simulink model "yinji"  (R2023a)
settings: Solver=VariableStepAuto  StartTime=0.0  StopTime=10.0  RelTol=1e-3
settings Model: Creator=Administrator  LastModifiedBy=Administrator

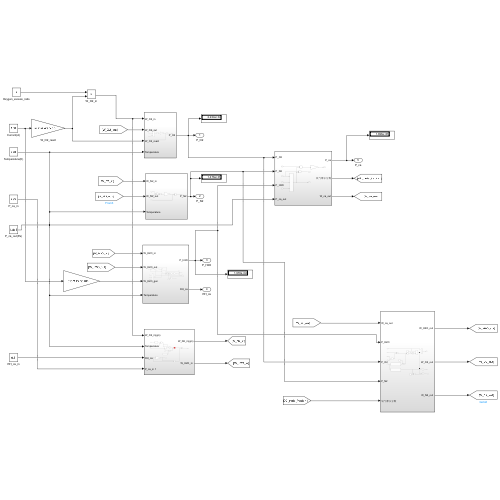
[thumbnail: Simulink's stored preview of the top-level diagram]
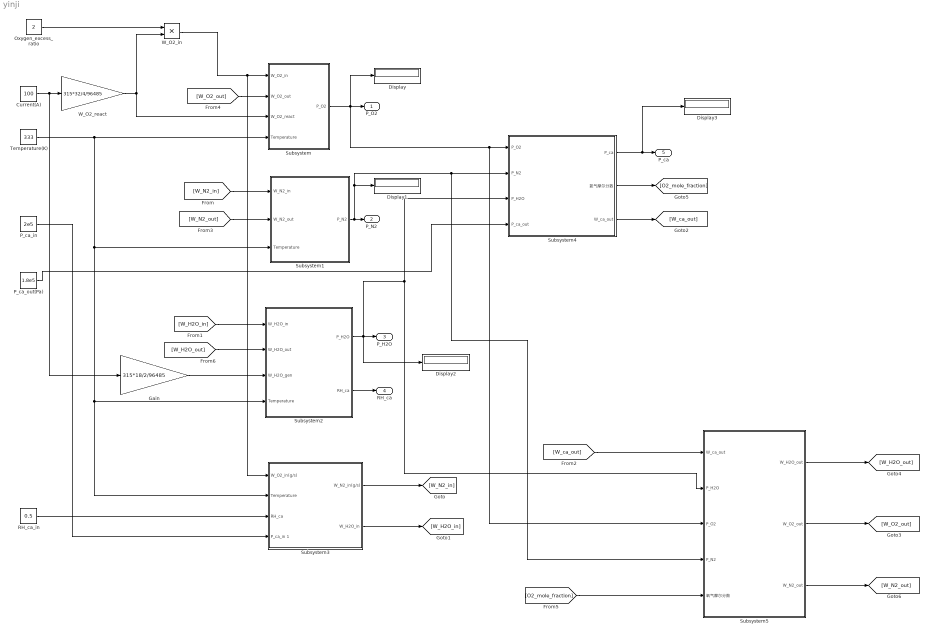
== system yinji ==
  Current(A) : Constant  Value=100
  Display{,1..3} (4 alike) : Display
  Gain : Gain  Gain=315*18/2/96485
  Oxygen_excess_ratio : Constant  Value=2
  P_ca_in : Constant  Value=2e5
  P_ca_out(Pa) : Constant  Value=1.8e5
  RH_ca_in : Constant  Value=0.5
  Subsystem : Subsystem
  Subsystem1 : Subsystem
  Subsystem2 : Subsystem
  Subsystem3 : Subsystem
  Subsystem4 : Subsystem
  Subsystem5 : Subsystem
  Temperature(K) : Constant  Value=333
  W_O2_in : Product
  W_O2_react : Gain  Gain=315*32/4/96485
  P_O2 : Outport
  P_N2 : Outport  Port=2
  P_H2O : Outport  Port=3
  RH_ca : Outport  Port=4
  P_ca : Outport  Port=5
  wires:
  [W_O2_out] -> Subsystem/2(W_O2_out)
  W_O2_react/1 -> W_O2_in/2, Subsystem/3(W_O2_react)
  Current(A)/1 -> Gain/1, W_O2_react/1
  Oxygen_excess_ratio/1 -> W_O2_in/1
  [W_N2_in] -> Subsystem1/1(W_N2_in)
  [W_N2_out] -> Subsystem1/2(W_N2_out)
  [W_H2O_in] -> Subsystem2/1(W_H2O_in)
  [W_H2O_out] -> Subsystem2/2(W_H2O_out)
  Gain/1 -> Subsystem2/3(W_H2O_gen)
  Subsystem2/2(RH_ca) -> RH_ca/1
  W_O2_in/1 -> Subsystem/1(W_O2_in), Subsystem3/1(W_O2_in(g/s))
  Temperature(K)/1 -> Subsystem2/4(Temperature), Subsystem3/2(Temperature), Subsystem1/3(Temperature), Subsystem/4(Temperature)
  RH_ca_in/1 -> Subsystem3/3("RH_ca ")
  P_ca_in/1 -> Subsystem3/4(P_ca_in 1)
  Subsystem3/1(W_N2_in(g/s)) -> [W_N2_in]
  Subsystem3/2("W_H2O_in ") -> [W_H2O_in]
  Subsystem1/1(P_N2) -> Display1/1, Subsystem5/4("P_N2 "), Subsystem4/2("P_N2 "), P_N2/1
  P_ca_out(Pa)/1 -> Subsystem4/4("P_ca_out ")
  Subsystem4/1(P_ca) -> Display3/1, P_ca/1
  Subsystem4/2(氧气摩尔分数) -> [O2_mole_fraction]
  Subsystem4/3(W_ca_out) -> [W_ca_out]
  [W_ca_out] -> Subsystem5/1("W_ca_out ")
  Subsystem2/1(P_H2O) -> Subsystem5/2("P_H2O "), Subsystem4/3("P_H2O "), Display2/1, P_H2O/1
  Subsystem/1(P_O2) -> Display/1, Subsystem5/3("P_O2 "), Subsystem4/1("P_O2 "), P_O2/1
  [O2_mole_fraction] -> Subsystem5/5("氧气摩尔分数 ")
  Subsystem5/1("W_H2O_out ") -> [W_H2O_out]
  Subsystem5/2("W_O2_out ") -> [W_O2_out]
  Subsystem5/3("W_N2_out ") -> [W_N2_out]

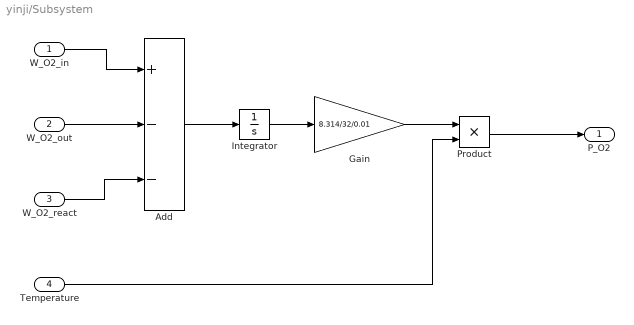
== system yinji/Subsystem ==
  W_O2_in : Inport
  W_O2_out : Inport  Port=2
  W_O2_react : Inport  Port=3
  Temperature : Inport  Port=4
  Add : Sum  Inputs=+--
  Gain : Gain  Gain=8.314/32/0.01
  Integrator : Integrator  InitialCondition=0.01
  Product : Product
  P_O2 : Outport
  wires:
  Temperature/1 -> Product/2
  Integrator/1 -> Gain/1
  Gain/1 -> Product/1
  W_O2_react/1 -> Add/3
  W_O2_in/1 -> Add/1
  Add/1 -> Integrator/1
  Product/1 -> P_O2/1
  W_O2_out/1 -> Add/2

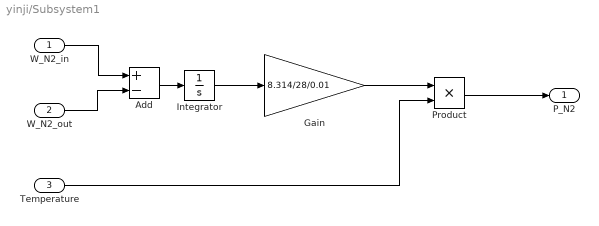
== system yinji/Subsystem1 ==
  W_N2_in : Inport
  W_N2_out : Inport  Port=2
  Temperature : Inport  Port=3
  Add : Sum  Inputs=+-
  Gain : Gain  Gain=8.314/28/0.01
  Integrator : Integrator  InitialCondition=0.01
  Product : Product
  P_N2 : Outport
  wires:
  Temperature/1 -> Product/2
  Integrator/1 -> Gain/1
  Product/1 -> P_N2/1
  Gain/1 -> Product/1
  W_N2_in/1 -> Add/1
  W_N2_out/1 -> Add/2
  Add/1 -> Integrator/1

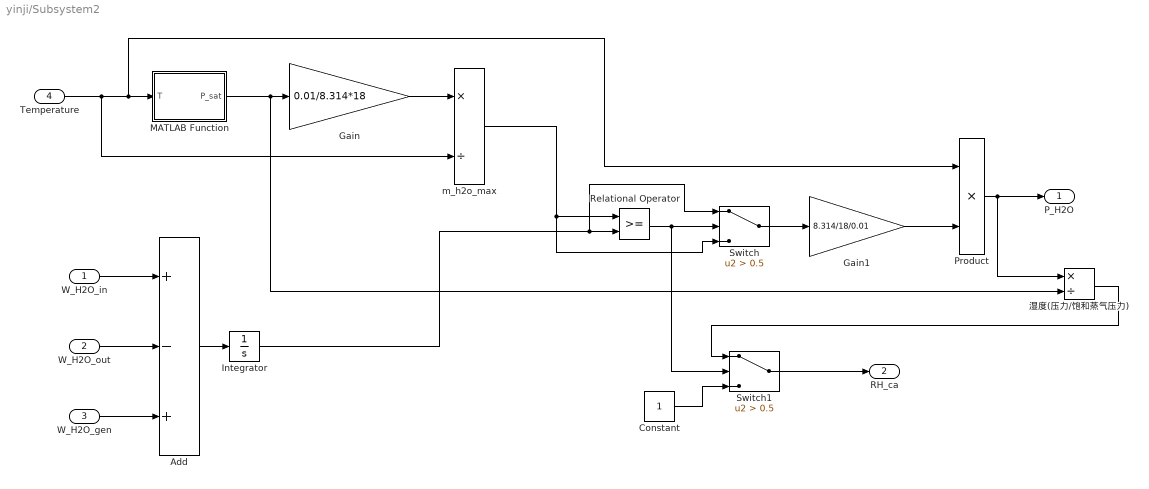
== system yinji/Subsystem2 ==
  W_H2O_in : Inport
  W_H2O_out : Inport  Port=2
  W_H2O_gen : Inport  Port=3
  Temperature : Inport  Port=4
  Add : Sum  Inputs=+-+
  Constant : Constant
  Gain : Gain  Gain=0.01/8.314*18
  Gain1 : Gain  Gain=8.314/18/0.01
  Integrator : Integrator  InitialCondition=0.01
  MATLAB Function : MATLAB Function  TreatAsAtomicUnit=on
  Product : Product
  Relational Operator : RelationalOperator  OutDataTypeStr=boolean  RndMeth=Simplest  InputSameDT=off
  Switch : Switch  Criteria=u2 > Threshold  Threshold=0.5  SaturateOnIntegerOverflow=off  InputSameDT=off
  Switch1 : Switch  Criteria=u2 > Threshold  Threshold=0.5  SaturateOnIntegerOverflow=off  InputSameDT=off
  m_h2o_max : Product  Inputs=*/
  湿度(压力/饱和蒸气压力) : Product  Inputs=*/
  P_H2O : Outport
  RH_ca : Outport  Port=2
  wires:
  湿度(压力/饱和蒸气压力)/1 -> Switch1/1
  Temperature/1 -> m_h2o_max/2, Product/1, MATLAB Function/1(T)
  W_H2O_in/1 -> Add/1
  W_H2O_gen/1 -> Add/3
  W_H2O_out/1 -> Add/2
  Gain1/1 -> Product/2
  Relational Operator/1 -> Switch1/2, Switch/2
  m_h2o_max/1 -> Relational Operator/1, Switch/3
  MATLAB Function/1(P_sat) -> 湿度(压力/饱和蒸气压力)/2, Gain/1
  Integrator/1 -> Switch/1, Relational Operator/2
  Constant/1 -> Switch1/3
  Switch/1 -> Gain1/1
  Add/1 -> Integrator/1
  Product/1 -> P_H2O/1, 湿度(压力/饱和蒸气压力)/1
  Gain/1 -> m_h2o_max/1
  Switch1/1 -> RH_ca/1

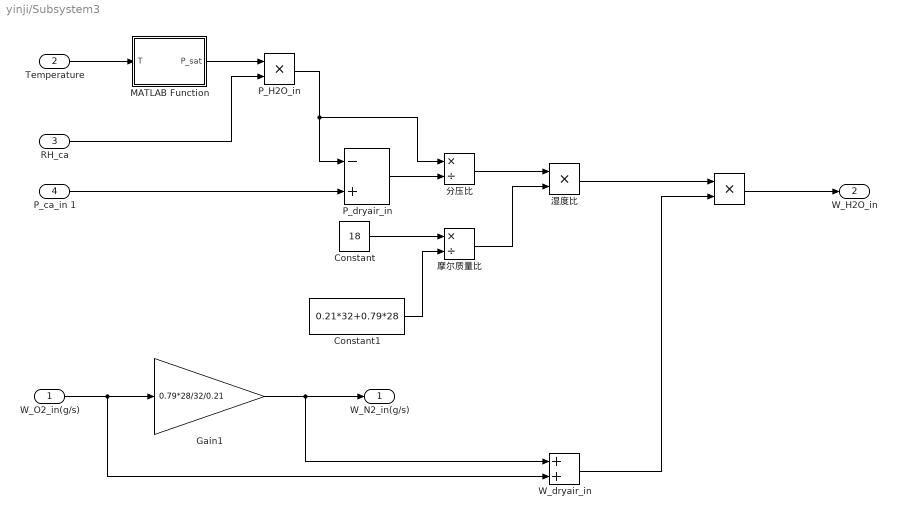
== system yinji/Subsystem3 ==
  W_O2_in(g/s) : Inport
  Temperature : Inport  Port=2
  "RH_ca " : Inport  Port=3
  P_ca_in 1 : Inport  Port=4
  "  " : Product
  Constant : Constant  Value=18
  Constant1 : Constant  Value=0.21*32+0.79*28
  Gain1 : Gain  Gain=0.79*28/32/0.21
  MATLAB Function : MATLAB Function  TreatAsAtomicUnit=on
  P_H2O_in : Product
  P_dryair_in : Sum  Inputs=-+
  W_dryair_in : Sum
  分压比 : Product  Inputs=*/
  摩尔质量比 : Product  Inputs=*/
  湿度比 : Product
  W_N2_in(g/s) : Outport
  "W_H2O_in " : Outport  Port=2
  wires:
  W_O2_in(g/s)/1 -> W_dryair_in/2, Gain1/1
  "  "/1 -> "W_H2O_in "/1
  "RH_ca "/1 -> P_H2O_in/2
  P_dryair_in/1 -> 分压比/2
  MATLAB Function/1(P_sat) -> P_H2O_in/1
  P_H2O_in/1 -> 分压比/1, P_dryair_in/1
  湿度比/1 -> "  "/1
  分压比/1 -> 湿度比/1
  W_dryair_in/1 -> "  "/2
  Temperature/1 -> MATLAB Function/1(T)
  P_ca_in 1/1 -> P_dryair_in/2
  Gain1/1 -> W_N2_in(g/s)/1, W_dryair_in/1
  Constant/1 -> 摩尔质量比/1
  Constant1/1 -> 摩尔质量比/2
  摩尔质量比/1 -> 湿度比/2

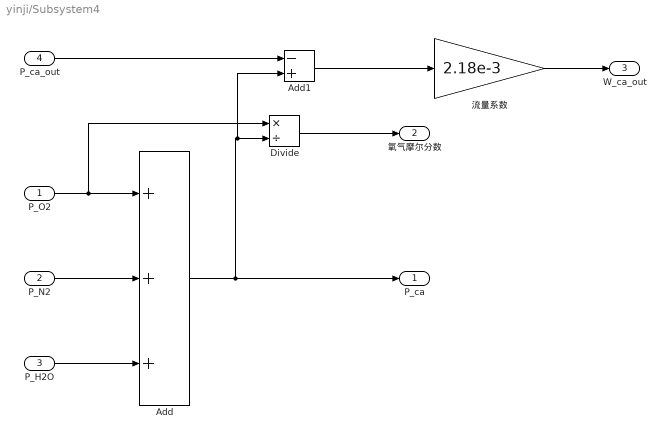
== system yinji/Subsystem4 ==
  "P_O2 " : Inport
  "P_N2 " : Inport  Port=2
  "P_H2O " : Inport  Port=3
  "P_ca_out " : Inport  Port=4
  Add : Sum  Inputs=+++
  Add1 : Sum  Inputs=-+
  Divide : Product  Inputs=*/
  流量系数 : Gain  Gain=2.18e-3
  P_ca : Outport
  氧气摩尔分数 : Outport  Port=2
  W_ca_out : Outport  Port=3
  wires:
  "P_ca_out "/1 -> Add1/1
  "P_O2 "/1 -> Divide/1, Add/1
  Add/1 -> P_ca/1, Add1/2, Divide/2
  Divide/1 -> 氧气摩尔分数/1
  Add1/1 -> 流量系数/1
  "P_N2 "/1 -> Add/2
  流量系数/1 -> W_ca_out/1
  "P_H2O "/1 -> Add/3

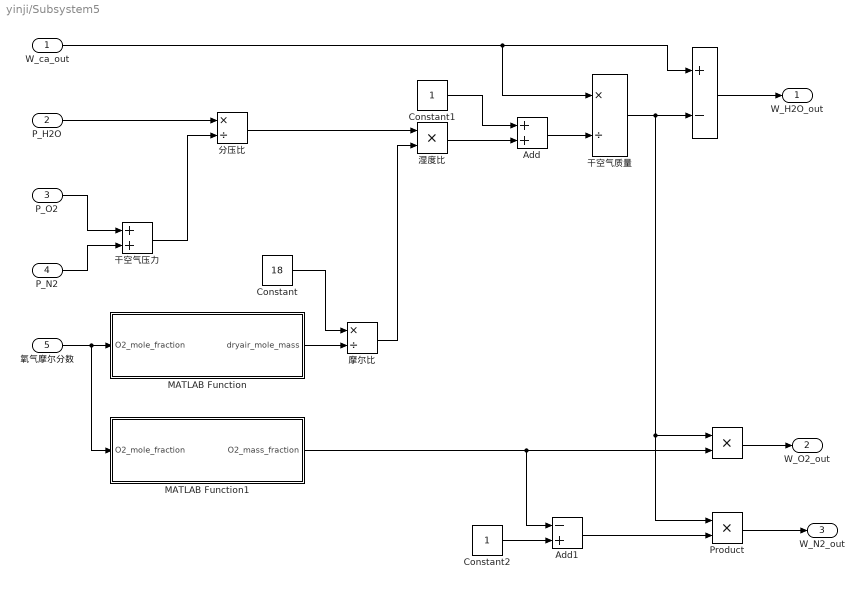
== system yinji/Subsystem5 ==
  "W_ca_out " : Inport
  "P_H2O " : Inport  Port=2
  "P_O2 " : Inport  Port=3
  "P_N2 " : Inport  Port=4
  "氧气摩尔分数 " : Inport  Port=5
  " " : Sum  Inputs=+-
  "  " : Product
  Add : Sum
  Add1 : Sum  Inputs=-+
  Constant : Constant  Value=18
  Constant1 : Constant
  Constant2 : Constant
  MATLAB Function : MATLAB Function  TreatAsAtomicUnit=on
  MATLAB Function1 : MATLAB Function  TreatAsAtomicUnit=on
  Product : Product
  分压比 : Product  Inputs=*/
  干空气压力 : Sum
  干空气质量 : Product  Inputs=*/
  摩尔比 : Product  Inputs=*/
  湿度比 : Product
  "W_H2O_out " : Outport
  "W_O2_out " : Outport  Port=2
  "W_N2_out " : Outport  Port=3
  wires:
  干空气压力/1 -> 分压比/2
  "P_O2 "/1 -> 干空气压力/1
  "W_ca_out "/1 -> " "/1, 干空气质量/1
  MATLAB Function1/1(O2_mass_fraction) -> Add1/1, "  "/2
  Add/1 -> 干空气质量/2
  Constant/1 -> 摩尔比/1
  湿度比/1 -> Add/2
  干空气质量/1 -> "  "/1, Product/1, " "/2
  摩尔比/1 -> 湿度比/2
  MATLAB Function/1(dryair_mole_mass) -> 摩尔比/2
  Constant1/1 -> Add/1
  分压比/1 -> 湿度比/1
  "氧气摩尔分数 "/1 -> MATLAB Function1/1(O2_mole_fraction), MATLAB Function/1(O2_mole_fraction)
  Constant2/1 -> Add1/2
  "  "/1 -> "W_O2_out "/1
  "P_N2 "/1 -> 干空气压力/2
  Product/1 -> "W_N2_out "/1
  Add1/1 -> Product/2
  " "/1 -> "W_H2O_out "/1
  "P_H2O "/1 -> 分压比/1

== matlab function yinji/Subsystem2/MATLAB Function ==
  data: T input; P_sat output
function P_sat = fcn(T)

P_sat = exp(23.196-3816.44/(T-46.13));

== matlab function yinji/Subsystem5/MATLAB Function ==
  data: O2_mole_fraction input; dryair_mole_mass output
function dryair_mole_mass= fcn(O2_mole_fraction)

dryair_mole_mass = O2_mole_fraction*32+(1-O2_mole_fraction)*28;

== matlab function yinji/Subsystem5/MATLAB Function1 ==
  data: O2_mole_fraction input; O2_mass_fraction output
function O2_mass_fraction= fcn(O2_mole_fraction)

O2_mass_fraction = O2_mole_fraction*32/(O2_mole_fraction*32+(1-O2_mole_fraction)*28);

== matlab function yinji/Subsystem3/MATLAB Function ==
  data: T input; P_sat output
function P_sat = fcn(T)

P_sat = exp(23.196-3816.44/(T-46.13));
